simulink model "boost_and_two_level_inverter_io_2_sc_ehs"  (R2021b)
settings: Solver=ode3  StartTime=0.0  StopTime=inf  FixedStep=2e-05  RelTol=1e-3
PostLoadFcn:
  | Boost_and_Two_Level_Inverter_param;
InitFcn:
  | Boost_and_Two_Level_Inverter_param;
undefined symbols (not defined in the file): Boost_PWM_Duty, Boost_PWM_Freq, Boost_Vin, Inv_BEMF_Ampl, Inv_PWM_CarrierFreq, Inv_PWM_ModulationIndex, Inv_PWM_Out, Inv_PWM_ShiftAngle
libraries: opal_lib x3
PreSaveFcn:
  | try, efsUpdateVersionAnnotation, end
settings Model: ARTEMISmethode_block_infos=$$__separator__$$  Creator=PYRobert  LastModifiedBy=ORTG
settings SolverCC: AlgebraicLoopSolver=TrustRegion
settings DataIOCC: LimitDataPoints=on  SaveFormat=Array  SignalLoggingSaveFormat=ModelDataLogs  SaveOutput=off  SignalLogging=off  SaveTime=off  ReturnWorkspaceOutputs=off  SignalLoggingName=sigsOut
settings OptimizationCC: BlockReduction=off  OptimizeBlockIOStorage=off  BufferReuse=off  GlobalBufferReuse=off  ExpressionFolding=off  ExpressionDepthLimit=2147483647  LocalBlockOutputs=off  InitFltsAndDblsToZero=on  LifeSpan=inf  OptimizeDataStoreBuffers=off  BusAssignmentInplaceUpdate=off
settings DebuggingCC: SaveWithParameterizedLinksMsg=none  UnderspecifiedInitializationDetection=Classic  MergeDetectMultiDrivingBlocksExec=none  SignalResolutionControl=TryResolveAllWithWarning  InheritedTsInSrcMsg=none  MultiTaskDSMMsg=warning  MultiTaskCondExecSysMsg=none  ParameterOverflowMsg=none  FcnCallInpInsideContextMsg=warning  StateNameClashWarn=warning  SFUnexpectedBacktrackingDiag=warning  SFNoUnconditionalDefaultTransitionDiag=warning  SFExecutionAtInitializationDiag=none  SFMachineParentedDataDiag=warning  ArithmeticOperatorsInVariantConditions=warning
settings HardwareCC: ProdBitPerPointer=32  ProdBitPerSizeT=32  ProdBitPerPtrDiffT=32  ProdLargestAtomicFloat=None  ProdIntDivRoundTo=Undefined  ProdEndianess=Unspecified  ProdWordSize=32  ProdHWDeviceType=32-bit Generic  TargetBitPerPointer=64  TargetBitPerSizeT=64  TargetBitPerPtrDiffT=64  TargetLongLongMode=on  TargetIntDivRoundTo=Zero  TargetEndianess=LittleEndian  TargetWordSize=64  TargetHWDeviceType=MATLAB Host  ProdEqTarget=off
settings ModelReferenceCC: PropagateSignalLabelsOutOfModel=off
settings SFSimCC: SimUseLocalCustomCode=off  CustomCodeUndefinedFunction=UseInterfaceOnly
settings RTWCC: GenCodeOnly=on  RTWUseLocalCustomCode=off
settings CodeAppCC: StateflowObjectComments=on
settings GRTTargetCC: TargetFcnLib=ansi_tfl_tmw.mat  TargetLangStandard=C89/C90 (ANSI)  CombineOutputUpdateFcns=off  GRTInterface=on
settings ConfigComp: CovMetricSettings=dw  CovSaveCumulativeToWorkspaceVar=on  CovSaveSingleToWorkspaceVar=on  CovExternalEMLEnable=off  CovSFcnEnable=off
settings SimscapeCC: SimscapeNormalizeSystem=off

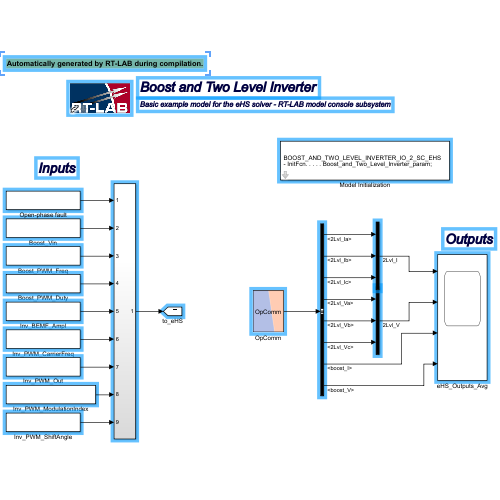
[thumbnail: Simulink's stored preview of the top-level diagram]
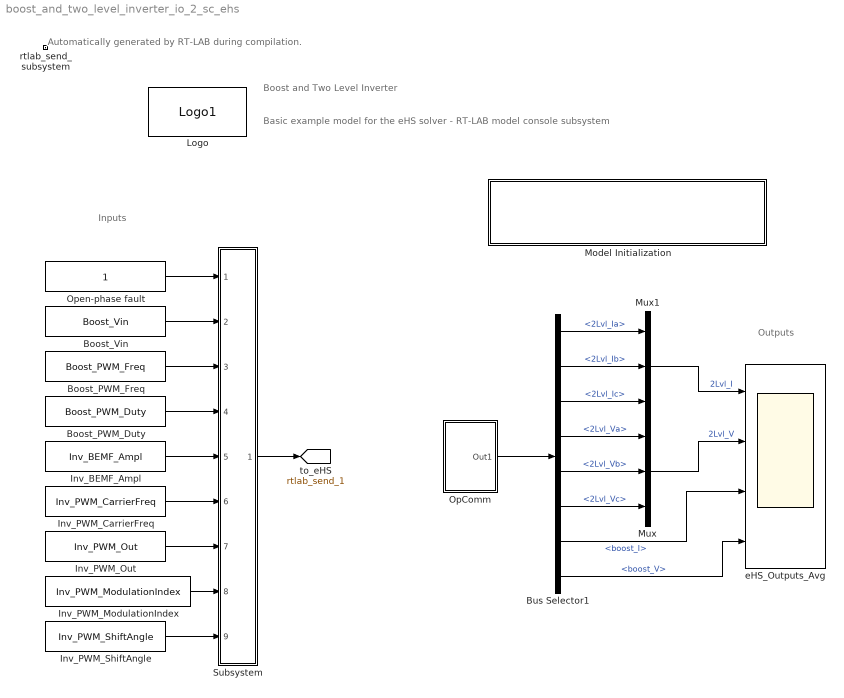
== system boost_and_two_level_inverter_io_2_sc_ehs ==
  note: Automatically generated by RT-LAB during compilation.
  note: Basic example model for the eHS solver - RT-LAB model console subsystem
  note: Boost and Two Level Inverter
  note: Outputs
  note: Inputs
  Boost_PWM_Duty : Constant  Value=Boost_PWM_Duty
  Boost_PWM_Freq : Constant  Value=Boost_PWM_Freq
  Boost_Vin : Constant  Value=Boost_Vin
  Bus Selector1 : BusSelector  OutputSignals=2Lvl_Ia,2Lvl_Ib,2Lvl_Ic,2Lvl_Va,2Lvl_Vb,2Lvl_Vc,boost_I,boost_V
  Inv_BEMF_Ampl : Constant  Value=Inv_BEMF_Ampl
  Inv_PWM_CarrierFreq : Constant  Value=Inv_PWM_CarrierFreq
  Inv_PWM_ModulationIndex : Constant  Value=Inv_PWM_ModulationIndex
  Inv_PWM_Out : Constant  Value=Inv_PWM_Out
  Inv_PWM_ShiftAngle : Constant  Value=Inv_PWM_ShiftAngle
  Logo : opal_lib/Logo1  vide=[]
  Model Initialization : Subsystem  mask(Model Functions){InitFcnX=Boost_and_Two_Level_Inverter_param;, prel=off, posl=on, inif=on, strf=off}
      mask prompts: InitFcnX "Initialisation"; prel "Preload Function"; posl "PostLoad Function"; inif "InitFcn"; strf "StartFcn"
      mask init:
      | currentBlock = gcb;
      | root = bdroot(currentBlock);
      | 
      | if ~strcmp(get_param(root,'BlockDiagramType'),'library')
      |     if prel==1
      |         set_param(root, 'PreLoadFcn', InitFcnX);
      |     else
      |         set_param(root, 'PreLoadFcn', '');
      |     end
      |     if inif==1
      |         set_param(root, 'InitFcn', InitFcnX);
      |     else
      |         set_param(root, 'InitFcn', '');
      |     end
      |     if strf==1
      |         set_param(root, 'StartFcn', InitFcnX);
      |     else
      |         set_param(root, 'StartFcn', '');
      |     end
      |     if posl==1
      |         set_param(root, 'PostLoadFcn', InitFcnX);
      |     else
      |         set_param(root, 'PostLoadFcn', '');
      |     end
      | end
      | 
      | pos = get_param(currentBlock, 'Position');
      | width = pos(3) - pos(1); height = pos(4) - pos(2);
      | txt = [ upper(root) '\n' '- InitFcn. . . . . '  get_param(root, 'InitFcn') ];
      settings: CopyFcn=set_param(gcb,'LinkStatus','none')
      mask Display: text(5, height*0.5, txt, 'horizontalAlignment', 'left', 'verticalAlignment', 'middle') ;
  Mux : Mux  Inputs=3
  Mux1 : Mux  Inputs=3
  OpComm : Subsystem
      mask init:
      | opmaskdisplay('maskdisplay_block',gcb,'disp(''OpComm'')');
      mask Display:
      | patch([0 0.5 0.7 0],[1 1 0 0],[0.7 0.75 0.9]);
      | patch([1 0.53 0.73 1],[1 1 0 0],[1 0.8 0.7]);
      | plot([0 0 1 1 0],[0 1 1 0 0]);
      | disp('OpComm')
  Open-phase fault : Constant
  Subsystem : Subsystem
  eHS_Outputs_Avg : Scope  NumInputPorts=4
  rtlab_send_subsystem : Subsystem  Priority=-100
      mask Display: text(0,0,'');
  tag scope: rtlab_send_1=global
  wires:
  Bus Selector1/7 -> eHS_Outputs_Avg/3  "<boost_I>"
  Mux/1 -> eHS_Outputs_Avg/2  "2Lvl_V"
  Bus Selector1/3 -> Mux1/3  "<2Lvl_Ic>"
  Bus Selector1/5 -> Mux/2  "<2Lvl_Vb>"
  Bus Selector1/8 -> eHS_Outputs_Avg/4  "<boost_V>"
  Bus Selector1/6 -> Mux/3  "<2Lvl_Vc>"
  Bus Selector1/4 -> Mux/1  "<2Lvl_Va>"
  Bus Selector1/2 -> Mux1/2  "<2Lvl_Ib>"
  Bus Selector1/1 -> Mux1/1  "<2Lvl_Ia>"
  Inv_PWM_ShiftAngle/1 -> Subsystem/9(In10)
  Mux1/1 -> eHS_Outputs_Avg/1  "2Lvl_I"
  OpComm/1(Out1) -> Bus Selector1/1
  Subsystem/1(Out1) -> [rtlab_send_1]
  Inv_PWM_ModulationIndex/1 -> Subsystem/8(In9)
  Inv_PWM_Out/1 -> Subsystem/7(In8)
  Inv_PWM_CarrierFreq/1 -> Subsystem/6(In7)
  Inv_BEMF_Ampl/1 -> Subsystem/5(In5)
  Boost_PWM_Duty/1 -> Subsystem/4(In4)
  Boost_PWM_Freq/1 -> Subsystem/3(In3)
  Boost_Vin/1 -> Subsystem/2(In2)
  Open-phase fault/1 -> Subsystem/1(In1)

== system boost_and_two_level_inverter_io_2_sc_ehs/Model Initialization ==

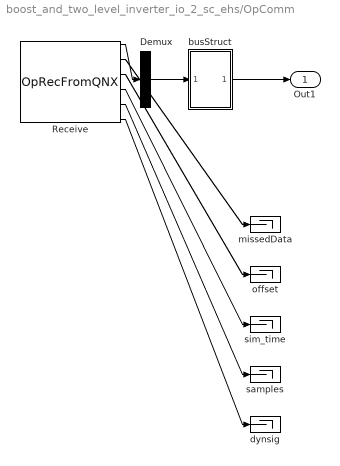
== system boost_and_two_level_inverter_io_2_sc_ehs/OpComm ==
  Demux : Demux  Outputs=[8]
  Receive : opal_lib/Communication/OpRecFromQNX  Node_num=1  Acqu_Group=1  Data_Width=8  Synchronization=off  Interpolation=off  Threshold=1.0  modelname=Boost_and_Two_Level_Inverter_IO  sampletime=2e-05
  busStruct : Subsystem
  dynsig : Terminator
  missedData : Terminator
  offset : Terminator
  samples : Terminator
  sim_time : Terminator
  Out1 : Outport
  wires:
  Demux/1 -> busStruct/1(In1)
  busStruct/1(Out1) -> Out1/1
  Receive/1 -> Demux/1
  Receive/6 -> dynsig/1
  Receive/5 -> samples/1
  Receive/4 -> sim_time/1
  Receive/3 -> offset/1
  Receive/2 -> missedData/1

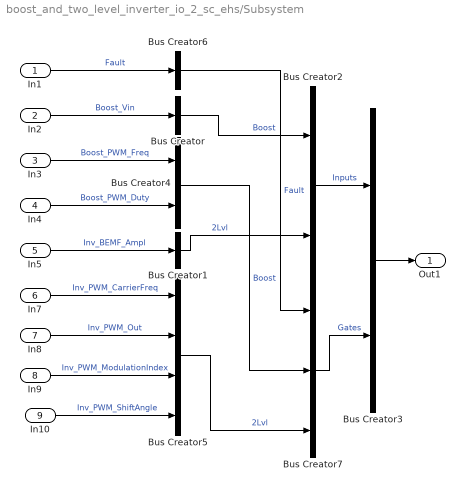
== system boost_and_two_level_inverter_io_2_sc_ehs/Subsystem ==
  In1 : Inport
  In2 : Inport  Port=2
  In3 : Inport  Port=3
  In4 : Inport  Port=4
  In5 : Inport  Port=5
  In7 : Inport  Port=6
  In8 : Inport  Port=7
  In9 : Inport  Port=8
  In10 : Inport  Port=9
  Bus Creator : BusCreator  Inputs=1
  Bus Creator1 : BusCreator  Inputs=1
  Bus Creator2 : BusCreator  Inputs=2
  Bus Creator3 : BusCreator  Inputs=2
  Bus Creator4 : BusCreator  Inputs=2
  Bus Creator5 : BusCreator  Inputs=4
  Bus Creator6 : BusCreator  Inputs=1
  Bus Creator7 : BusCreator  Inputs=3
  Out1 : Outport  VectorParamsAs1DForOutWhenUnconnected=off
  wires:
  In4/1 -> Bus Creator4/2  "Boost_PWM_Duty"
  Bus Creator2/1 -> Bus Creator3/1  "Inputs"
  Bus Creator1/1 -> Bus Creator2/2  "2Lvl"
  In8/1 -> Bus Creator5/2  "Inv_PWM_Out"
  In5/1 -> Bus Creator1/1  "Inv_BEMF_Ampl"
  In1/1 -> Bus Creator6/1  "Fault"
  In2/1 -> Bus Creator/1  "Boost_Vin"
  Bus Creator/1 -> Bus Creator2/1  "Boost"
  Bus Creator7/1 -> Bus Creator3/2  "Gates"
  In9/1 -> Bus Creator5/3  "Inv_PWM_ModulationIndex"
  Bus Creator4/1 -> Bus Creator7/2  "Boost"
  In3/1 -> Bus Creator4/1  "Boost_PWM_Freq"
  In7/1 -> Bus Creator5/1  "Inv_PWM_CarrierFreq"
  Bus Creator3/1 -> Out1/1
  Bus Creator6/1 -> Bus Creator7/1  "Fault"
  Bus Creator5/1 -> Bus Creator7/3  "2Lvl"
  In10/1 -> Bus Creator5/4  "Inv_PWM_ShiftAngle"

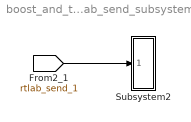
== system boost_and_two_level_inverter_io_2_sc_ehs/rtlab_send_subsystem ==
  Subsystem2 : Subsystem
  wires:
  [rtlab_send_1] -> Subsystem2/1(In1)

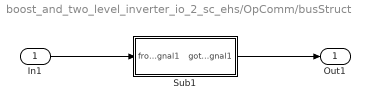
== system boost_and_two_level_inverter_io_2_sc_ehs/OpComm/busStruct ==
  In1 : Inport
  Sub1 : Subsystem
  Out1 : Outport
  wires:
  Sub1/1(goto_signal1) -> Out1/1
  In1/1 -> Sub1/1(from_signal1)

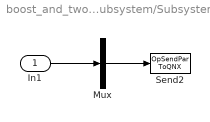
== system boost_and_two_level_inverter_io_2_sc_ehs/rtlab_send_subsystem/Subsystem2 ==
  In1 : Inport  PortDimensions=9
  Mux : Mux  Inputs=1
  Send2 : opal_lib/Communication/OpSendPar ToQNX  Node_num=1  modelname=Boost_and_Two_Level_Inverter_IO
  wires:
  Mux/1 -> Send2/1
  In1/1 -> Mux/1

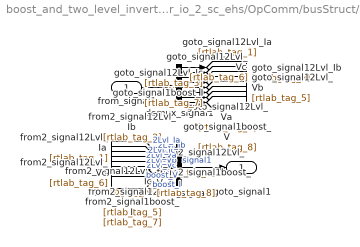
== system boost_and_two_level_inverter_io_2_sc_ehs/OpComm/busStruct/Sub1 ==
  from_signal1 : Inport
  buscre_signal1 : BusCreator  Inputs=8
  demux_signal1 : Demux  Outputs="[1  1  1  1  1  1  1  1]"
  goto_signal1 : Outport
  wires:
  buscre_signal1/1 -> goto_signal1/1  "signal1"
  [rtlab_tag_8] -> buscre_signal1/8  "boost_V"
  [rtlab_tag_7] -> buscre_signal1/7  "boost_I"
  [rtlab_tag_6] -> buscre_signal1/6  "2Lvl_Vc"
  [rtlab_tag_5] -> buscre_signal1/5  "2Lvl_Vb"
  [rtlab_tag_4] -> buscre_signal1/4  "2Lvl_Va"
  [rtlab_tag_3] -> buscre_signal1/3  "2Lvl_Ic"
  [rtlab_tag_2] -> buscre_signal1/2  "2Lvl_Ib"
  [rtlab_tag_1] -> buscre_signal1/1  "2Lvl_Ia"
  demux_signal1/8 -> [rtlab_tag_8]
  demux_signal1/7 -> [rtlab_tag_7]
  demux_signal1/6 -> [rtlab_tag_6]
  demux_signal1/5 -> [rtlab_tag_5]
  demux_signal1/4 -> [rtlab_tag_4]
  demux_signal1/3 -> [rtlab_tag_3]
  demux_signal1/2 -> [rtlab_tag_2]
  demux_signal1/1 -> [rtlab_tag_1]
  from_signal1/1 -> demux_signal1/1
